simulink model "L22MSDsim"  (R2020a)
settings: Solver=FixedStepAuto  StartTime=0.0  StopTime=10  FixedStep=0.001  RelTol=1e-3
InitFcn:
  | L22MSDparameters;
values from neighbouring files (symbols this model uses):
  A = [0 1 ; -k/m -b/m]    [L22MSDparameters.m]
  B = [0 ; 1/m]    [L22MSDparameters.m]
  C = [1 0]    [L22MSDparameters.m]
  KLQR = lqr(A,B,Q,R)    [L22MSDparameters.m]
  x0 = [1; 0.5]    [L22MSDparameters.m]
  x0hat = [x0(1); 0]    [L22MSDparameters.m]
undefined symbols (not defined in the file or in its folder): LKB
libraries: simulink x1
settings Model: Creator=vcichella  LastModifiedBy=vcichella

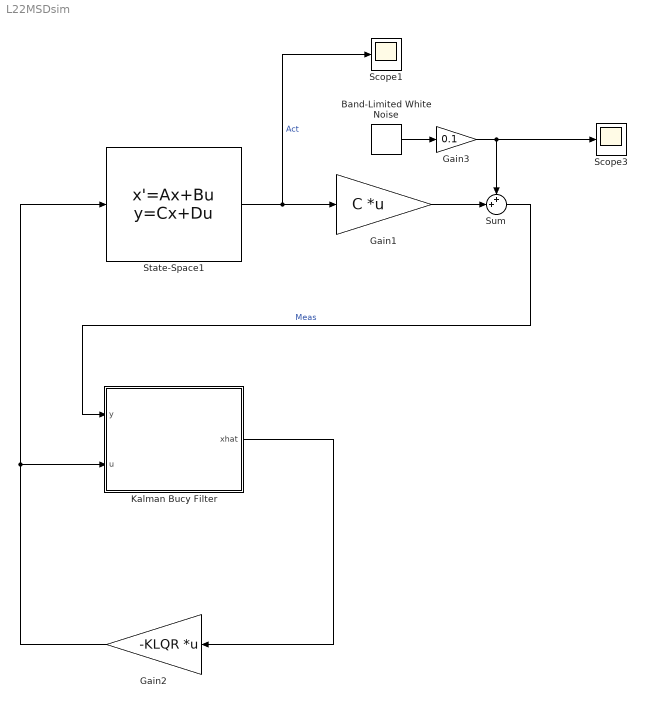
== system L22MSDsim ==
  Band-Limited White Noise : simulink/Sources/Band-Limited White Noise  Cov=[0.01]  Ts=0.01  seed=[23341]
  Gain1 : Gain  Gain=C  Multiplication=Matrix(K*u)
  Gain2 : Gain  Gain=-KLQR  Multiplication=Matrix(K*u)
  Gain3 : Gain  Gain=0.1
  Kalman Bucy Filter : Subsystem
  Scope1 : Scope
  Scope3 : Scope
  State-Space1 : StateSpace  A=A  B=B  C=eye(size(A))  D=zeros(2,1)  InitialCondition=x0
  Sum : Sum  Inputs=++|
  wires:
  State-Space1/1 -> Scope1/1, Gain1/1  "Act"
  Kalman Bucy Filter/1(xhat) -> Gain2/1
  Sum/1 -> Kalman Bucy Filter/1(y)  "Meas"
  Gain1/1 -> Sum/2
  Band-Limited White Noise/1 -> Gain3/1
  Gain2/1 -> State-Space1/1, Kalman Bucy Filter/2(u)
  Gain3/1 -> Sum/1, Scope3/1

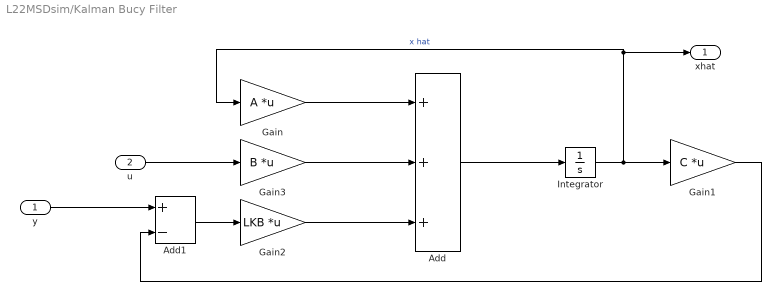
== system L22MSDsim/Kalman Bucy Filter ==
  y : Inport
  u : Inport  Port=2
  Add : Sum  Inputs=+++
  Add1 : Sum  Inputs=+-
  Gain : Gain  Gain=A  Multiplication=Matrix(K*u)
  Gain1 : Gain  Gain=C  Multiplication=Matrix(K*u)
  Gain2 : Gain  Gain=LKB  Multiplication=Matrix(K*u)
  Gain3 : Gain  Gain=B  Multiplication=Matrix(K*u)
  Integrator : Integrator  InitialCondition=x0hat
  xhat : Outport
  wires:
  Gain3/1 -> Add/2
  u/1 -> Gain3/1
  Gain2/1 -> Add/3
  y/1 -> Add1/1
  Add1/1 -> Gain2/1
  Gain1/1 -> Add1/2
  Gain/1 -> Add/1
  Add/1 -> Integrator/1
  Integrator/1 -> Gain1/1, Gain/1, xhat/1  "x hat"
